simulink model "ac2dc_motor_driver"  (R2018a)
settings: Solver=ode23tb  StartTime=0.0  StopTime=10  MaxStep=1e-4  RelTol=1e-4
libraries: powerlib x17, powerlib_meascontrol x1
settings Model: Creator=Caner  LastModifiedBy=bulbu
settings OptimizationCC: LifeSpan=inf
settings DebuggingCC: SFExecutionAtInitializationDiag=none
settings CodeAppCC: StateflowObjectComments=on
settings SimscapeCC: SimscapeNormalizeSystem=off

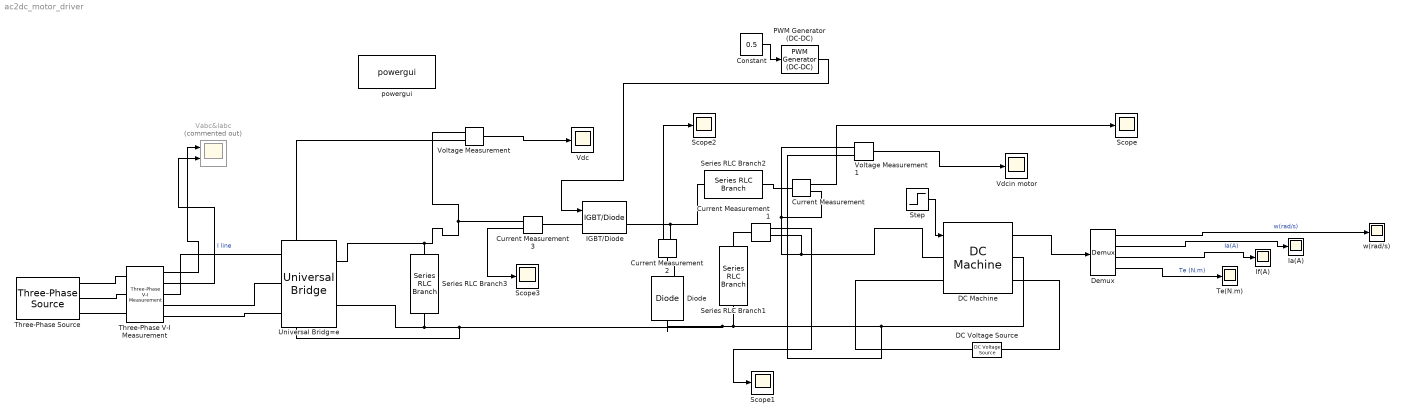
== system ac2dc_motor_driver ==
  Constant : Constant  Value=0.5
  Current Measurement{,1..3} (4 alike) : powerlib/Measurements/Current Measurement  PhasorSimulation=off  OutputType=Complex  PSBequivalent=0
  DC Machine : powerlib/Machines/DC Machine  PresetModel=No  MechanicalLoad=Torque TL  FieldType=Wound  ShowDetailedParameters=on  MeasurementBus=off  RLa="[ 1.07  24.5e-3]"  RLf="[ 210  23]"  Laf=2  MachineConstant=Torque constant (N.m/A)  Ke=1.8  Kt=1.8  J=1  Bm=0  Tf=0  w0=1  Ifinit=1  TsPowergui=0  TsBlock=-1
  DC Voltage Source : powerlib/Electrical Sources/DC Voltage Source  Amplitude=125  Measurements=None
  Demux : Demux
  Diode : powerlib/Power Electronics/Diode  Ron=0.001  Lon=0  Vf=0.8  IC=0  UseSnubber=0  Rs=inf  Cs=inf  Measurements=on
  IGBT/Diode : powerlib/Power Electronics/IGBT//Diode  Ron=1e-3  Rs=inf  Cs=inf  Measurements=on
  Ia(A) : Scope
  If(A) : Scope
  PWM Generator (DC-DC) : powerlib_meascontrol/Pulse & Signal Generators/PWM Generator (DC-DC)  Fsw=976  Ts=0
  Scope{,1..3} (4 alike) : Scope
  Series RLC Branch1 : powerlib/Elements/Series RLC Branch  LConnTagsString=__new0  RConnTagsString=__new0  BranchType=C  Resistance=1  Inductance=1e-3  SetiL0=off  InitialCurrent=0  Capacitance=470e-6  Setx0=off  InitialVoltage=0  Measurements=None
  Series RLC Branch2 : powerlib/Elements/Series RLC Branch  LConnTagsString=__new0  RConnTagsString=__new0  BranchType=L  Resistance=1  Inductance=10e-3  SetiL0=off  InitialCurrent=0  Capacitance=1e-3  Setx0=off  InitialVoltage=0  Measurements=None
  Series RLC Branch3 : powerlib/Elements/Series RLC Branch  LConnTagsString=__new0  RConnTagsString=__new0  BranchType=C  Resistance=1  Inductance=1e-3  SetiL0=off  InitialCurrent=0  Capacitance=660e-6  Setx0=off  InitialVoltage=0  Measurements=None
  Step : Step  Time=0.1  After=25  SampleTime=0
  Te(N.m) : Scope
  Three-Phase V-I Measurement : powerlib/Measurements/Three-Phase V-I Measurement  VoltageMeasurement=phase-to-ground  SetLabelV=off  LabelV=Vabc  Vpu=off  VpuLL=off  CurrentMeasurement=yes  SetLabelI=off  LabelI=Iabc  Ipu=off  Pbase=100e6  Vbase=500e3  OutputType=Complex  PhasorSimulation=off  PSBequivalent=0
  Three-Phase Source : powerlib/Electrical Sources/Three-Phase Source  InternalConnection=Yg  VoltagePhases=off  Voltage=160  PhaseAngle=0  Voltage_phases=[25e3 25e3 25e3]/sqrt(3)  PhaseAngles_phases=[0 -120 +120]  Frequency=50  NonIdealSource=on  SpecifyImpedance=off  Resistance=0.1  Inductance=100e-6  ShortCircuitLevel=100e6  BaseVoltage=180  XRratio=7  BusType=swing  Pref=10e3  Qref=0  Prefabc=[10e3, 10e3, 10e3]  Qrefabc=[0, 0, 0]  Qmin=-inf  Qmax=inf
  Universal Bridg=e : powerlib/Power Electronics/Universal Bridge  Arms=3  SnubberResistance=inf  SnubberCapacitance=inf  Device=Diodes  Ron=20e-3  Lon=0  ForwardVoltages="[  0  0  ]"  ForwardVoltage=0.575  GTOparameters=[ 10e-6 , 20e-6 ]  IGBTparameters=[ 1e-6 , 2e-6 ]  Measurements=All voltages and currents  Measurements_2=None  converterType=Rectifier
  Vabc&Iabc : Scope  Commented=on  NumInputPorts=2
  "Vdc " : Scope
  Vdcin motor : Scope
  Voltage Measurement : powerlib/Measurements/Voltage Measurement  PhasorSimulation=off  OutputType=Complex  PSBequivalent=0
  Voltage Measurement1 : powerlib/Measurements/Voltage Measurement  PhasorSimulation=off  OutputType=Complex  PSBequivalent=0
  powergui : powerlib/powergui  Priority=1  SimulationMode=Continuous  SampleTime=50e-6  frequency=60  Iterations=50  frequencyindice=0  Pbase=100e6  ErrMax=1e-4  UnitsV=kV  UnitsW=MW  buscounter=0  FunctionMessages=off  echomessages=off  EnableUseOfTLC=off  CurrentSourceSwitches=off  DisableSnubberDevices=off  DisableRonSwitches=off  DisableVfSwitches=off  DisplayEquations=off  SolverType=Tustin/Backward Euler (TBE)  Interpol=off  ExternalGateDelay=off  methode=off  Ts=100  x0status=blocks  SPID=on  SwTol=0  HookPort=off  RestoreLinks=warning  ResistiveCurrentMeasurement=off  Frange=[0:2:500]  Ylog=off  Xlog=on  ShowGrid=off  save=off  variable=ZData  structure=0  ZoomFFT=off  StartTime=0.0  cycles=1  DisplayStyle=1  fundamental=60  FreqAxis=off  MaxFrequency=1000  frequencyindicesteady=1  RmsSteady=1  display=off
  w(rad/s) : Scope
  wires:
  Three-Phase V-I Measurement/2 -> Vabc&Iabc/2  "I line"
  Three-Phase V-I Measurement/1 -> Vabc&Iabc/1
  Demux/2 -> Ia(A)/1  "Ia(A)"
  Demux/1 -> w(rad/s)/1  "w(rad/s)"
  DC Machine/1 -> Demux/1
  Demux/3 -> If(A)/1
  Demux/4 -> Te(N.m)/1  "Te (N.m)"
  Voltage Measurement/1 -> "Vdc "/1
  Voltage Measurement1/1 -> Vdcin motor/1
  Step/1 -> DC Machine/1
  Constant/1 -> PWM Generator (DC-DC)/1
  Current Measurement/1 -> Scope/1
  Current Measurement1/1 -> Scope1/1
  Current Measurement2/1 -> Scope2/1
  Current Measurement3/1 -> Scope3/1
  PWM Generator (DC-DC)/1 -> IGBT/Diode/1
  connections:
  Three-Phase Source/RConn3 -- Three-Phase V-I Measurement/LConn3
  Three-Phase V-I Measurement/RConn1 -- Universal Bridg=e/LConn1
  Three-Phase Source/RConn1 -- Three-Phase V-I Measurement/LConn1
  Three-Phase Source/RConn2 -- Three-Phase V-I Measurement/LConn2
  Three-Phase V-I Measurement/RConn2 -- Universal Bridg=e/LConn2
  Three-Phase V-I Measurement/RConn3 -- Universal Bridg=e/LConn3
  Voltage Measurement/LConn1 -- Current Measurement3/RConn1 -- Series RLC Branch3/LConn1 -- Universal Bridg=e/RConn1
  DC Voltage Source/RConn1 -- DC Machine/LConn2
  IGBT/Diode/RConn1 -- Series RLC Branch2/RConn1 -- Current Measurement2/RConn1
  Universal Bridg=e/RConn2 -- Voltage Measurement1/LConn2 -- DC Machine/RConn1 -- Series RLC Branch1/RConn1 -- Diode/LConn1 -- Voltage Measurement/LConn2 -- Series RLC Branch3/RConn1
  Series RLC Branch2/LConn1 -- Current Measurement/LConn1
  DC Machine/LConn1 -- Current Measurement1/RConn1 -- Current Measurement/RConn1 -- Voltage Measurement1/LConn1
  Current Measurement1/LConn1 -- Series RLC Branch1/LConn1
  Diode/RConn1 -- Current Measurement2/LConn1
  Current Measurement3/LConn1 -- IGBT/Diode/LConn1
  DC Voltage Source/LConn1 -- DC Machine/RConn2
